simulink model "Hss_buckboost_det_20250602"  (R2024b)
settings: Solver=VariableStepAuto  StartTime=0.0  StopTime=0.2  RelTol=1e-3
StartFcn:
  | tic
StopFcn:
  | toc
values from neighbouring files (symbols this model uses):
  Af = mtoeplitz(A)    [HSS_buckboost_ave_20250528.m]    (also in HSS_buckboost_det_20250528.m; param_BuckboostHSS_ave_simulink_20250604.m; param_BuckboostHSS_det_simulink_20250602.m)
  alpha = 5/17    (= 0.294117647059)    [HSS_buckboost_ave_20250528.m]    (also in HSS_buckboost_det_20250528.m; param_BuckboostHSS_ave_simulink_20250604.m; param_BuckboostHSS_det_simulink_20250602.m)
  Bf = mtoeplitz(B)    [HSS_buckboost_ave_20250528.m]    (also in HSS_buckboost_det_20250528.m; param_BuckboostHSS_ave_simulink_20250604.m; param_BuckboostHSS_det_simulink_20250602.m)
  C = 3.55*10^-3    (= 0.00355)    [HSS_buckboost_ave_20250528.m]    (also in HSS_buckboost_det_20250528.m; param_BuckboostHSS_ave_simulink_20250604.m; param_BuckboostHSS_det_simulink_20250602.m)
  fft_sw_N = (conj(fft_sw_N))    [HSS_buckboost_det_20250528.m]    (also in param_BuckboostHSS_det_simulink_20250602.m = fft_sw_N')
  Fnom = 50    [HSS_buckboost_ave_20250528.m]    (also in HSS_buckboost_det_20250528.m; param_BuckboostHSS_ave_simulink_20250604.m; param_BuckboostHSS_det_simulink_20250602.m)
  L = length(t)    [HSS_buckboost_ave_20250528.m]    (also in HSS_buckboost_det_20250528.m; param_BuckboostHSS_ave_simulink_20250604.m; param_BuckboostHSS_det_simulink_20250602.m)
  N = 30    [HSS_buckboost_ave_20250528.m]    (also in HSS_buckboost_det_20250528.m; param_BuckboostHSS_ave_simulink_20250604.m; param_BuckboostHSS_det_simulink_20250602.m)
  Nt = blkdiag(Nt,1i*w0*k*I)    [HSS_buckboost_ave_20250528.m]    (also in HSS_buckboost_det_20250528.m; param_BuckboostHSS_ave_simulink_20250604.m; param_BuckboostHSS_det_simulink_20250602.m)
  R = 3.57    [HSS_buckboost_ave_20250528.m]    (also in HSS_buckboost_det_20250528.m; param_BuckboostHSS_ave_simulink_20250604.m; param_BuckboostHSS_det_simulink_20250602.m)
  Ts = 1e-7    (= 1e-07)    [HSS_buckboost_ave_20250528.m]    (also in HSS_buckboost_det_20250528.m; param_BuckboostHSS_ave_simulink_20250604.m; param_BuckboostHSS_det_simulink_20250602.m)
  Vin = 12    [HSS_buckboost_ave_20250528.m]    (also in HSS_buckboost_det_20250528.m; param_BuckboostHSS_ave_simulink_20250604.m; param_BuckboostHSS_det_simulink_20250602.m)
libraries: spsCurrentMeasurementLib x3, spsSeriesRLCBranchLib x3, spsMosfetLib x2, spsDCVoltageSourceLib x1, spsDiodeLib x1, spsGroundLib x1, eePwmGenerator x1, spsVoltageMeasurementLib x1, sps_lib x1, spspowerguiLib x1
settings Model: Creator=DELL  LastModifiedBy=ana
settings OptimizationCC: ReuseModelBlockBuffer=off
settings RTWCC: GPUComputeCapability=3.5

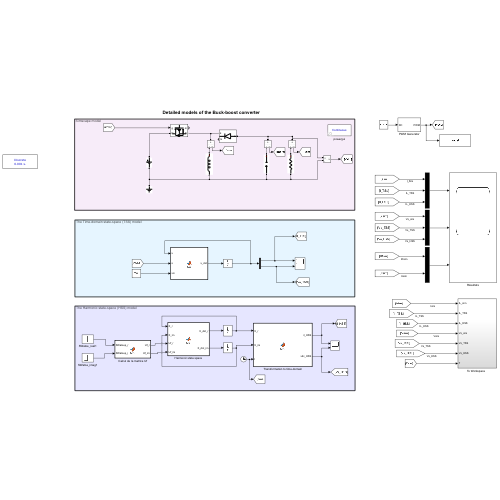
[thumbnail: Simulink's stored preview of the top-level diagram]
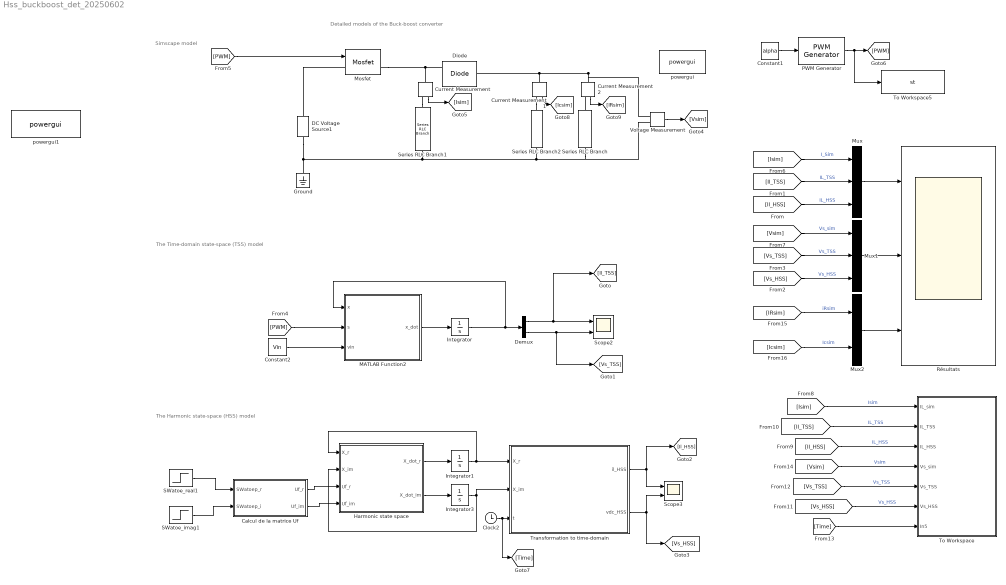
== system Hss_buckboost_det_20250602 ==
  note: Simscape model
  note: The Harmonic state-space (HSS) model
  note: The Time-domain state-space (TSS) model
  note: Detailed models of the Buck-boost converter
  Calcul de la matrice Uf : MATLAB Function  TreatAsAtomicUnit=on
  Clock2 : Clock
  Constant1 : Constant  Value=alpha
  Constant2 : Constant  Value=Vin
  Current Measurement : spsCurrentMeasurementLib/Current Measurement  PhasorSimulation=off  OutputType=Complex  PSBequivalent=0
  Current Measurement1 : spsCurrentMeasurementLib/Current Measurement  PhasorSimulation=off  OutputType=Complex  PSBequivalent=0
  Current Measurement2 : spsCurrentMeasurementLib/Current Measurement  PhasorSimulation=off  OutputType=Complex  PSBequivalent=0
  DC Voltage Source1 : spsDCVoltageSourceLib/DC Voltage Source  Amplitude=Vin  Measurements=None
  Demux : Demux  Outputs=2
  Diode : spsDiodeLib/Diode  Ron=0  Lon=0  Vf=0  IC=0  UseSnubber=0  Rs=inf  Cs=0  Measurements=on
  Ground : spsGroundLib/Ground  LConnTagsString=a
  Harmonic state space : MATLAB Function  TreatAsAtomicUnit=on
  Integrator : Integrator
  Integrator1 : Integrator
  Integrator3 : Integrator
  MATLAB Function2 : MATLAB Function  TreatAsAtomicUnit=on
  Mosfet : spsMosfetLib/Mosfet  Ron=0.001  Lon=0  Rd=0  Vfd=0  IC=0  Rs=inf  Cs=0  Measurements=on
  Mux : Mux  Inputs=3
  Mux1 : Mux  Inputs=3
  Mux2 : Mux  Inputs=2
  PWM Generator : eePwmGenerator/PWM Generator  CarrCount=Up  Tper=0.01  Tdelay=0  Ts=5e-5
  Résultats : Scope  NumInputPorts=3
  SWatoe_imag1 : Step  Time=0  Before=imag(fft_sw_N)  After=imag(fft_sw_N)  SampleTime=Ts
  SWatoe_real1 : Step  Time=0  Before=real(fft_sw_N)  After=real(fft_sw_N)  SampleTime=Ts
  Scope2 : Scope  NumInputPorts=2
  Scope3 : Scope  NumInputPorts=2
  Series RLC Branch : spsSeriesRLCBranchLib/Series RLC Branch  LConnTagsString=__new0  RConnTagsString=__new0  BranchType=R  Resistance=R  Inductance=1e-3  SetiL0=off  InitialCurrent=0  Capacitance=1e-6  Setx0=off  InitialVoltage=0  Measurements=None
  Series RLC Branch1 : spsSeriesRLCBranchLib/Series RLC Branch  LConnTagsString=__new0  RConnTagsString=__new0  BranchType=L  Resistance=0  Inductance=L  SetiL0=off  InitialCurrent=0  Capacitance=1e-6  Setx0=off  InitialVoltage=0  Measurements=None
  Series RLC Branch2 : spsSeriesRLCBranchLib/Series RLC Branch  LConnTagsString=__new0  RConnTagsString=__new0  BranchType=C  Resistance=1  Inductance=1e-3  SetiL0=off  InitialCurrent=0  Capacitance=C  Setx0=off  InitialVoltage=0  Measurements=None
  "To Workspace   " : Subsystem
  To Workspace5 : ToWorkspace  VariableName=st  SaveFormat=Structure With Time  SampleTime=-1
  Transformation to time-domain : MATLAB Function  TreatAsAtomicUnit=on
  Voltage Measurement : spsVoltageMeasurementLib/Voltage Measurement  PhasorSimulation=off  OutputType=Complex  PSBequivalent=0
  powergui : sps_lib/powergui  Priority=1  SimulationMode=Continuous  SampleTime=50e-6  frequency=60  Iterations=50  frequencyindice=0  Pbase=100e6  ErrMax=1e-4  UnitsV=kV  UnitsW=MW  buscounter=0  FunctionMessages=off  echomessages=off  EnableUseOfTLC=off  CurrentSourceSwitches=off  DisableSnubberDevices=off  DisableRonSwitches=off  DisableVfSwitches=off  DisplayEquations=off  AutomaticDiscreteSolvers=off  SolverType=Tustin/Backward Euler (TBE)  Interpol=off  ExternalGateDelay=off  methode=off  Ts=100  x0status=blocks  SPID=on  SwTol=0  HookPort=off  NonlinearTolerance=1e-4  nMaxIteration=100  ContinueOnMaxIteration=off  RestoreLinks=warning  ResistiveCurrentMeasurement=off  Frange=[0:2:500]  Ylog=off  Xlog=on  ShowGrid=off  save=off  variable=ZData  structure=0  ZoomFFT=off  StartTime=0.0  cycles=1  DisplayStyle=1  fundamental=60  FreqAxis=off  MaxFrequency=1000  frequencyindicesteady=1  RmsSteady=1  display=off
  powergui1 : spspowerguiLib/powergui  SimulationMode=Discrete  SampleTime=Ts  frequency=60  Iterations=50  frequencyindice=0  Pbase=100e6  ErrMax=1e-4  UnitsV=kV  UnitsW=MW  buscounter=0  FunctionMessages=off  echomessages=off  EnableUseOfTLC=off  CurrentSourceSwitches=off  DisableSnubberDevices=off  DisableRonSwitches=off  DisableVfSwitches=off  DisplayEquations=off  AutomaticDiscreteSolvers=off  SolverType=Tustin/Backward Euler (TBE)  Interpol=off  ExternalGateDelay=off  methode=off  Ts=0  x0status=blocks  SPID=off  SwTol=0  HookPort=off  NonlinearTolerance=1e-4  nMaxIteration=100  ContinueOnMaxIteration=off  RestoreLinks=warning  ResistiveCurrentMeasurement=off  Frange=[0:2:500]  Ylog=off  Xlog=on  ShowGrid=off  save=off  variable=ZData  structure=ta_loic  ZoomFFT=off  StartTime=0.12  cycles=1  DisplayStyle=2  fundamental=60  FreqAxis=on  MaxFrequency=100000  frequencyindicesteady=1  RmsSteady=1  display=off
  wires:
  Demux/1 -> [Il_TSS], Scope2/1
  PWM Generator/1 -> To Workspace5/1, [PWM]
  MATLAB Function2/1(x_dot) -> Integrator/1
  Demux/2 -> [Vs_TSS], Scope2/2
  Constant2/1 -> MATLAB Function2/3(vin)
  Constant1/1 -> PWM Generator/1
  Integrator/1 -> MATLAB Function2/1(x), Demux/1
  Clock2/1 -> [Time], Transformation to time-domain/3(t)
  Calcul de la matrice Uf/2(Uf_im) -> Harmonic state space/4(Uf_im)
  Calcul de la matrice Uf/1(Uf_r) -> Harmonic state space/3(Uf_r)
  Integrator3/1 -> Harmonic state space/2(X_im), Transformation to time-domain/2(X_im)
  Integrator1/1 -> Transformation to time-domain/1(X_r), Harmonic state space/1(X_r)
  Transformation to time-domain/1(il_HSS) -> Scope3/1, [Il_HSS]
  SWatoe_real1/1 -> Calcul de la matrice Uf/1(SWatoep_r)
  Transformation to time-domain/2(vdc_HSS) -> [Vs_HSS], Scope3/2
  Harmonic state space/1(X_dot_r) -> Integrator1/1
  Harmonic state space/2(X_dot_im) -> Integrator3/1
  SWatoe_imag1/1 -> Calcul de la matrice Uf/2(SWatoep_i)
  Voltage Measurement/1 -> [Vsim]
  [PWM] -> MATLAB Function2/2(s)
  [PWM] -> Mosfet/1
  [Isim] -> Mux/1  "I_Sim"
  [Il_TSS] -> Mux/2  "IL_TSS"
  [Il_HSS] -> Mux/3  "IL_HSS"
  Mux/1 -> Résultats/1
  [Vsim] -> Mux1/1  "Vs_sim"
  Mux1/1 -> Résultats/2
  [Vs_TSS] -> Mux1/2  "Vs_TSS"
  [Vs_HSS] -> Mux1/3  "Vs_HSS"
  [Vs_HSS] -> "To Workspace   "/6(Vs_HSS)  "Vs_HSS"
  [Il_TSS] -> "To Workspace   "/2(IL_TSS)  "IL_TSS"
  [Vs_TSS] -> "To Workspace   "/5(Vs_TSS)  "Vs_TSS"
  [Il_HSS] -> "To Workspace   "/3(IL_HSS)  "IL_HSS"
  [Time] -> "To Workspace   "/7(In5)
  [Isim] -> "To Workspace   "/1(IL_sim)  "Isim"
  [Vsim] -> "To Workspace   "/4(Vs_sim)  "Vsim"
  Current Measurement/1 -> [Isim]
  Current Measurement1/1 -> [Icsim]
  Current Measurement2/1 -> [IRsim]
  [IRsim] -> Mux2/1  "iRsim"
  [Icsim] -> Mux2/2  "Icsim"
  Mux2/1 -> Résultats/3
  connections:
  Ground/LConn1 -- Series RLC Branch1/RConn1 -- Series RLC Branch/RConn1 -- Voltage Measurement/LConn2 -- Series RLC Branch2/RConn1 -- DC Voltage Source1/LConn1
  DC Voltage Source1/RConn1 -- Mosfet/LConn1
  Mosfet/RConn1 -- Current Measurement/LConn1 -- Diode/RConn1
  Voltage Measurement/LConn1 -- Current Measurement2/LConn1 -- Current Measurement1/LConn1 -- Diode/LConn1
  Current Measurement/RConn1 -- Series RLC Branch1/LConn1
  Current Measurement1/RConn1 -- Series RLC Branch2/LConn1
  Series RLC Branch/LConn1 -- Current Measurement2/RConn1

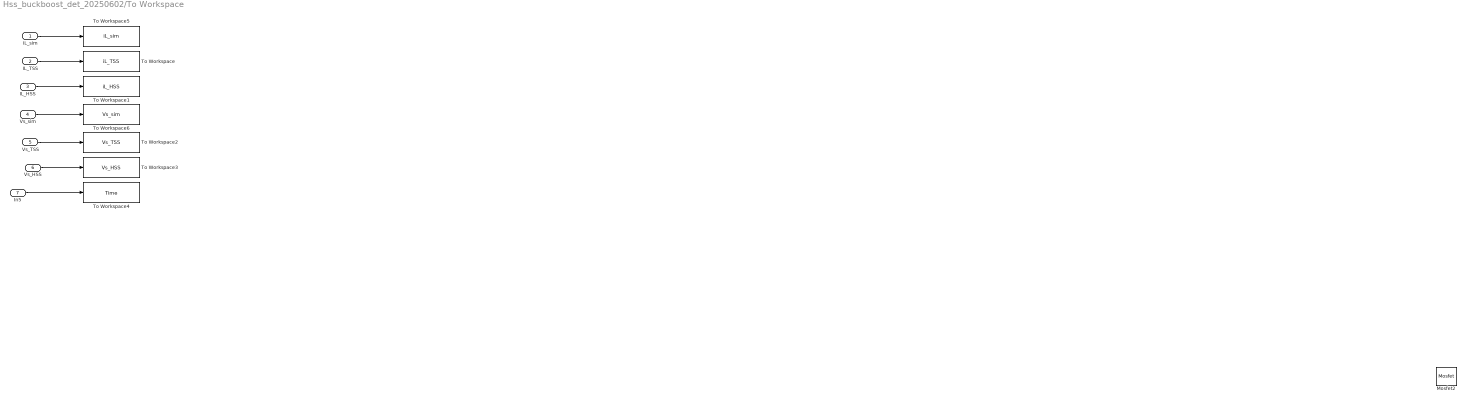
== system Hss_buckboost_det_20250602/To Workspace    ==
  IL_sim : Inport
  IL_TSS : Inport  Port=2
  IL_HSS : Inport  Port=3
  Vs_sim : Inport  Port=4
  Vs_TSS : Inport  Port=5
  Vs_HSS : Inport  Port=6
  In5 : Inport  Port=7
  Mosfet2 : spsMosfetLib/Mosfet  Ron=0.1  Lon=0  Rd=0.01  Vfd=0  IC=0  Rs=1e5  Cs=inf  Measurements=on
  To Workspace : ToWorkspace  VariableName=iL_TSS  SampleTime=-1
  To Workspace1 : ToWorkspace  VariableName=iL_HSS  SampleTime=-1
  To Workspace2 : ToWorkspace  VariableName=Vs_TSS  SampleTime=-1
  To Workspace3 : ToWorkspace  VariableName=Vs_HSS  SampleTime=-1
  To Workspace4 : ToWorkspace  VariableName=Time  SampleTime=-1
  To Workspace5 : ToWorkspace  VariableName=iL_sim  SampleTime=-1
  To Workspace6 : ToWorkspace  VariableName=Vs_sim  SampleTime=-1
  wires:
  IL_TSS/1 -> To Workspace/1
  In5/1 -> To Workspace4/1
  IL_HSS/1 -> To Workspace1/1
  Vs_HSS/1 -> To Workspace3/1
  Vs_TSS/1 -> To Workspace2/1
  IL_sim/1 -> To Workspace5/1
  Vs_sim/1 -> To Workspace6/1

== matlab function Hss_buckboost_det_20250602/Transformation to time-domain ==
  data: X_r input size=[(2*N+1)*2,1]; X_im input size=[(2*N+1)*2,1]; t input; il_HSS output; vdc_HSS output; N parameter; Fnom parameter
function [il_HSS,vdc_HSS] = fcn(X_r,X_im,t,N, Fnom)

w0 = 2*pi*Fnom;

Xss = X_r+1i*X_im;

%% Restitution of vectors from Xss
Il = zeros(2*N+1,1);
Vs = zeros(2*N+1,1);
v = [Il,Vs];     % Matrix composed by the Fourier coefficients
v_r=[Il,Vs];
v_i=[Il,Vs];

for i = 1:size(v,2)
    j = i;
    k = 1;                 
    while j <= (2*N+1)*2
        v_r(k,i) = real(Xss(j));
        v_i(k,i) = imag(Xss(j));
        j = j+2;
        k = k+1;
    end
end

v=v_r+1i*v_i;
gamma = 0;

for k = -N:N
    if k==-N
        gamma = exp(w0*k*1i*t);
    else
        gamma = [gamma, exp(w0*k*1i*t)];
    end
end

il_HSS = real(gamma*v(:,1)); % il(t) = sum_k=-N:N( Il_k . exp(+w0*k*1i*t) )
vdc_HSS = real(gamma*v(:,2)); % Vs(t) = sum_k=-N:N( Vs_k . exp(+w0*k*1i*t) )

== matlab function Hss_buckboost_det_20250602/Calcul de la matrice Uf ==
  data: Uf_r output size=[(2*N+1),1]; R parameter; C parameter; L parameter; Vin parameter; Uf_im output size=[(2*N+1),1]; SWatoep_r input size=[2*N+1,1]; SWatoep_i input
function [Uf_r ,Uf_im] = fcn(R, C, L, Vin, SWatoep_r,SWatoep_i)

SWatoep = SWatoep_r + 1i*SWatoep_i;

Uf=Vin*SWatoep;

Uf_r = real(Uf);
Uf_im = imag(Uf);

== matlab function Hss_buckboost_det_20250602/MATLAB Function2 ==
  data: x input size=[2,1]; x_dot output; s input; vin input; L parameter; C parameter; R parameter

function x_dot  = fcn(x, s, vin,L, C, R)

il = x(1);
vs = x(2);

sw =s;

il_dot = ((sw/L)*vin+((1-sw)/L)*vs);

vs_dot = (((sw-1)/C)*il+(-1/(R*C))*vs);

x_dot = [il_dot;vs_dot];

== matlab function Hss_buckboost_det_20250602/Harmonic state space ==
  settings: updateMethod=CONTINUOUS  sampleTime=Ts
  data: X_r input size=[(2*N+1)*2,1]; X_im input size=[(2*N+1)*2,1]; Uf_r input size=[(2*N+1),1]; Uf_im input size=[(2*N+1),1]; X_dot_r output size=[(2*N+1)*2,1]; X_dot_im output size=[(2*N+1)*2,1]; Af parameter; Bf parameter; Nt parameter
function [X_dot_r,X_dot_im]  = fcn(X_r, X_im,Uf_r, Uf_im, Af,Bf,Nt)
X=X_r+1i*X_im;

Uf=Uf_r+1i*Uf_im;
X_dot=(Af-Nt)*X+Bf*Uf;

X_dot_r=real(X_dot);
X_dot_im=imag(X_dot);
